simulink model "moonlander_parametrized"  (R2016a)
settings: Solver=ode4  StartTime=0.0  StopTime=100.0  FixedStep=0.01  RelTol=1e-3
model workspace (MAT data in the model file):
  End1 = 10
  End2 = 10
  Start1 = 1
  Start2 = 1
settings Model: Creator=s1710595017  LastModifiedBy=Peter
settings DataIOCC: ExternalInput=[Start1, End1, Start2, End2]  LoadExternalInput=on  SaveFormat=Array
settings OptimizationCC: LifeSpan=1
settings DebuggingCC: SFUnexpectedBacktrackingDiag=error  SFNoUnconditionalDefaultTransitionDiag=error
settings GRTTargetCC: TargetLangStandard=C99 (ISO)  GeneratePreprocessorConditionals=Use local settings
settings ConfigComp: CovMetricSettings=dwe  CovHtmlReporting=off  CovSaveCumulativeToWorkspaceVar=off  CovSaveSingleToWorkspaceVar=off  CovExternalEMLEnable=on

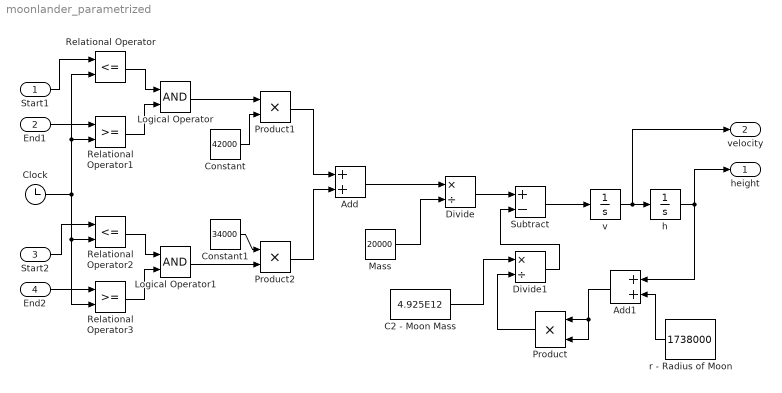
== system moonlander_parametrized ==
  Start1 : Inport
  End1 : Inport  Port=2
  Start2 : Inport  Port=3
  End2 : Inport  Port=4
  Add : Sum
  Add1 : Sum
  "C2 - Moon Mass " : Constant  Value=4.925E12
  Clock : Clock
  Constant : Constant  Value=42000
  Constant1 : Constant  Value=34000
  Divide : Product  Inputs=*/
  Divide1 : Product  Inputs=*/
  Logical Operator : Logic  AllPortsSameDT=off  OutDataTypeStr=boolean
  Logical Operator1 : Logic  AllPortsSameDT=off  OutDataTypeStr=boolean
  Mass : Constant  Value=20000
  Product : Product
  Product1 : Product
  Product2 : Product
  Relational Operator : RelationalOperator  Operator=<=  OutDataTypeStr=boolean
  Relational Operator1 : RelationalOperator  OutDataTypeStr=boolean
  Relational Operator2 : RelationalOperator  Operator=<=  OutDataTypeStr=boolean
  Relational Operator3 : RelationalOperator  OutDataTypeStr=boolean
  Subtract : Sum  Inputs=+-
  h : Integrator  InitialCondition=1000
  r - Radius of Moon : Constant  Value=1738000
  v : Integrator  InitialCondition=-10
  height : Outport
  velocity : Outport  Port=2
  wires:
  Product/1 -> Divide1/2
  r - Radius of Moon/1 -> Add1/2
  Subtract/1 -> v/1
  "C2 - Moon Mass "/1 -> Divide1/1
  Divide/1 -> Subtract/1
  Add1/1 -> Product/2, Product/1
  Divide1/1 -> Subtract/2
  Product1/1 -> Add/1
  Add/1 -> Divide/1
  v/1 -> velocity/1, h/1
  Mass/1 -> Divide/2
  h/1 -> height/1, Add1/1
  Product2/1 -> Add/2
  Start1/1 -> Relational Operator/1
  End1/1 -> Relational Operator1/1
  Relational Operator/1 -> Logical Operator/1
  Relational Operator1/1 -> Logical Operator/2
  Logical Operator/1 -> Product1/1
  Relational Operator2/1 -> Logical Operator1/1
  Logical Operator1/1 -> Product2/2
  Relational Operator3/1 -> Logical Operator1/2
  Start2/1 -> Relational Operator2/1
  Clock/1 -> Relational Operator3/2, Relational Operator2/2, Relational Operator1/2, Relational Operator/2
  End2/1 -> Relational Operator3/1
  Constant/1 -> Product1/2
  Constant1/1 -> Product2/1
